simulink model "speedbackword"  (R2016b)
settings: Solver=VariableStepAuto  StartTime=0.0  StopTime=20  RelTol=1e-3
libraries: simulink x2
settings Model: Creator=CYC  LastModifiedBy=CYC

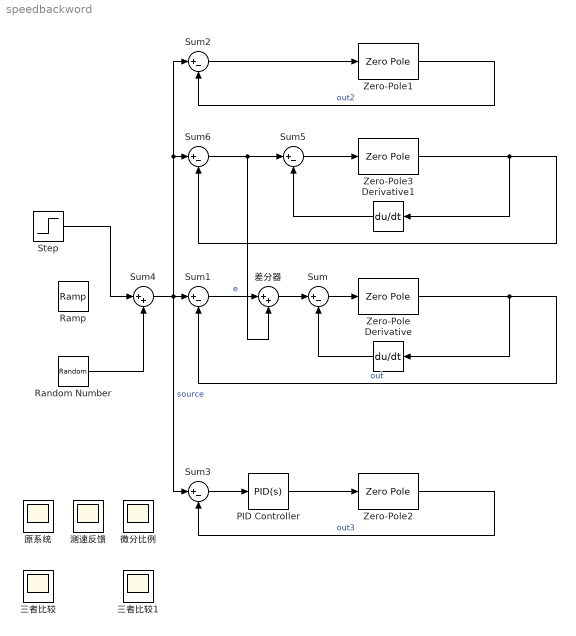
== system speedbackword ==
  Derivative : Derivative  CoefficientInTFapproximation=0.22
  Derivative1 : Derivative  CoefficientInTFapproximation=0.22
  PID Controller : simulink/Continuous/PID Controller  Controller=PID  TimeDomain=Continuous-time  SampleTime=-1  IntegratorMethod=Forward Euler  FilterMethod=Forward Euler  Form=Parallel  UseFilter=on  ControllerParametersSource=internal  P=5  I=0  D=0.38  N=100  InitialConditionSource=internal  InitialConditionForIntegrator=0  InitialConditionForFilter=0  ExternalReset=none  LimitOutput=off  UpperSaturationLimit=inf  LowerSaturationLimit=-inf  LinearizeAsGain=on  AntiWindupMode=none  Kb=1  TrackingMode=off  Kt=1  PParamMin=[]  PParamMax=[]  IParamMin=[]  IParamMax=[]  DParamMin=[]  DParamMax=[]  NParamMin=[]  NParamMax=[]  KbParamMin=[]  KbParamMax=[]  KtParamMin=[]  KtParamMax=[]  POutMin=[]  POutMax=[]  IOutMin=[]  IOutMax=[]  DOutMin=[]  DOutMax=[]  NOutMin=[]  NOutMax=[]  KbOutMin=[]  KbOutMax=[]  KtOutMin=[]  KtOutMax=[]  IntegratorOutMin=[]  IntegratorOutMax=[]  FilterOutMin=[]  FilterOutMax=[]  SumOutMin=[]  SumOutMax=[]  SumI1OutMin=[]  SumI1OutMax=[]  SumI2OutMin=[]  SumI2OutMax=[]  SumI3OutMin=[]  SumI3OutMax=[]  SumDOutMin=[]  SumDOutMax=[]  SaturationOutMin=[]  SaturationOutMax=[]  IntegratorContinuousStateAttributes=''  IntegratorStateMustResolveToSignalObject=off  IntegratorRTWStateStorageClass=Auto  FilterContinuousStateAttributes=''  FilterStateMustResolveToSignalObject=off  FilterRTWStateStorageClass=Auto  DifferentiatorICPrevScaledInput=0  DifferentiatorOutMin=[]  DifferentiatorOutMax=[]
  Ramp : simulink/Sources/Ramp  slope=1  start=0  X0=0
  Random Number : RandomNumber  SampleTime=0.1
  Step : Step  After=10  SampleTime=0
  Sum{,1..3,5..6} (6 alike) : Sum  Inputs=|+-
  Sum4 : Sum  Inputs=|++
  Zero-Pole{,1..3} (4 alike) : ZeroPole  Zeros=[]  Poles=[0 -1]  Gain=[10]
  三者比较 : Scope
      settings: Floating=on
  三者比较1 : Scope
      settings: Floating=on
  原系统 : Scope
      settings: Floating=on
  差分器 : Sum  Inputs=|++
  "微分比例 " : Scope
      settings: Floating=on
  测速反馈 : Scope
      settings: Floating=on
  wires:
  Zero-Pole/1 -> Derivative/1, Sum1/2  "out"
  Derivative/1 -> Sum/2
  Sum/1 -> Zero-Pole/1
  Sum2/1 -> Zero-Pole1/1
  Zero-Pole1/1 -> Sum2/2  "out2"
  Zero-Pole2/1 -> Sum3/2  "out3"
  PID Controller/1 -> Zero-Pole2/1
  Sum3/1 -> PID Controller/1
  Sum4/1 -> Sum3/1, Sum1/1, Sum6/1, Sum2/1  "source"
  Zero-Pole3/1 -> Derivative1/1, Sum6/2
  Derivative1/1 -> Sum5/2
  Sum5/1 -> Zero-Pole3/1
  Sum6/1 -> 差分器/2, Sum5/1
  差分器/1 -> Sum/1
  Sum1/1 -> 差分器/1  "e"
  Step/1 -> Sum4/1
  Random Number/1 -> Sum4/2
